simulink model "sf_cdplayer"  (Simulink 7.6)
settings: Solver=FixedStepDiscrete  StartTime=0.0  StopTime=inf  FixedStep=1  RelTol=1e-3
PreLoadFcn:
  | defaultRadioRequestMode = RadioRequestMode.OFF;
  | defaultCdRequestMode = CdRequestMode.EMPTY;
StartFcn:
  | clear sfcdplayerhelper;
  | sfcdplayergui;
StopFcn:
  | delete(sfcdplayergui);
model workspace (MATLAB code in the model file):
  | Ts = 0.01;  % setup system sample rate
settings Model: Creator=The MathWorks Inc.
settings DataIOCC: SaveOutput=off  SaveTime=off
settings OptimizationCC: InlineParams=on  StateBitsets=on  DataBitsets=on  ZeroExternalMemoryAtStartup=off  ZeroInternalMemoryAtStartup=off  InitFltsAndDblsToZero=on  EfficientFloat2IntCast=on  EfficientMapNaN2IntZero=off  OptimizeModelRefInitCode=on  LifeSpan=1
settings DebuggingCC: SolverPrmCheckMsg=none  StrictBusMsg=Warning
settings HardwareCC: ProdIntDivRoundTo=Zero  ProdEndianess=LittleEndian  ProdHWDeviceType=NEC->V850
settings ModelReferenceCC: ModelReferenceNumInstancesAllowed=Single
settings SFSimCC: SimParseCustomCode=off
settings RTWCC: SystemTargetFile=ert.tlc  GenCodeOnly=on  TemplateMakefile=ert_default_tmf  Description=Real-Time Workshop Embedded Coder (no auto configuration)  GenerateReport=on  ProcessScript=ert_make_rtw_hook  IncludeHyperlinkInReport=on  LaunchReport=on  GenerateTraceInfo=on  GenerateTraceReport=on  GenerateTraceReportSl=on  GenerateTraceReportSf=on  GenerateTraceReportEml=on
settings CodeAppCC: IgnoreCustomStorageClasses=off
settings ERTTargetCC: MultiwordLength=2048  GenerateSampleERTMain=on  IncludeMdlTerminateFcn=off  SupportAbsoluteTime=off  SupportNonFinite=off  SupportComplex=off  PurelyIntegerCode=on  ERTCustomFileTemplate=example_file_process.tlc  ConvertIfToSwitch=off  EnableUserReplacementTypes=on
settings ConfigComp: Description=Design Verifier Custom Configuration Component  DVMaxProcessTime=600  DVDisplayUnsatisfiableObjectives=on  DVAutomaticStubbing=off  DVParameters=on  DVModelCoverageObjectives=MCDC  DVMaxTestCaseSteps=500  DVTestSuiteOptimization=CombinedObjectives  DVSaveHarnessModel=on  DVModelReferenceHarness=on  DVSaveReport=on

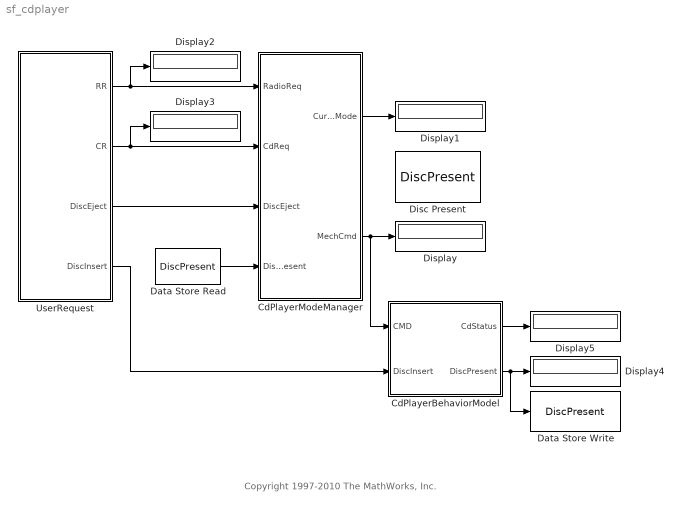
== system sf_cdplayer ==
  note: Copyright 1997-2010 The MathWorks, Inc.
  CdPlayerBehaviorModel : Stateflow chart  TreatAsAtomicUnit=on
  CdPlayerModeManager : Stateflow chart  TreatAsAtomicUnit=on
  Data Store Read : DataStoreRead  DataStoreName=DiscPresent  SampleTime=0
  Data Store Write : DataStoreWrite  DataStoreName=DiscPresent
  Disc Present : DataStoreMemory  DataStoreName=DiscPresent
  Display{,1..5} (6 alike) : Display
  UserRequest : Stateflow chart  TreatAsAtomicUnit=on
  wires:
  UserRequest/2(CR) -> CdPlayerModeManager/2(CdReq), Display3/1
  Data Store Read/1 -> CdPlayerModeManager/4(DiscPresent)
  CdPlayerModeManager/2(MechCmd) -> Display/1, CdPlayerBehaviorModel/1(CMD)
  CdPlayerModeManager/1(CurrentRadioMode) -> Display1/1
  UserRequest/1(RR) -> CdPlayerModeManager/1(RadioReq), Display2/1
  CdPlayerBehaviorModel/1(CdStatus) -> Display5/1
  CdPlayerBehaviorModel/2(DiscPresent) -> Data Store Write/1, Display4/1
  UserRequest/4(DiscInsert) -> CdPlayerBehaviorModel/2(DiscInsert)
  UserRequest/3(DiscEject) -> CdPlayerModeManager/3(DiscEject)

== stateflow chart CdPlayerModeManager ==
  state Eject
    entry:
    MechCmd = EJECT;
  state ModeManager
    (history)
    state ON
      (history)
      state FMMode
        entry:
        CurrentRadioMode = FM;
        MechCmd = STOP;
      state CDMode
        en:
        CurrentRadioMode = CD;
        MechCmd = STOP;
        ex: MechCmd = STOP;
        state Play
          state FastForward
            entry: MechCmd = FF;
          state Rew
            entry: MechCmd = REW;
          state Normal
            entry: MechCmd = PLAY;
          Play -> FastForward [order 1] : [CdReq == FF && !in(FastForward)]
          (default) -> Normal
          Play -> Rew [order 2] : [CdReq == REW && !in(Rew)]
          Play -> Normal [order 3] : [CdReq == PLAY && !in(Normal)]
        state Stop
          entry: MechCmd = STOP;
        (default) -> Stop [order 2]
        (default) -> Play [order 1] : [DiscPresent]
        Play -> Stop [order 1] : [CdReq==STOP]
        Stop -> Play : [DiscPresent && CdReq==PLAY]
      state AMMode
        entry:
        CurrentRadioMode = AM;
        MechCmd = STOP;
      (junction 17) -> AMMode [order 1] : [RadioReq==AM]
      (junction 15) -> FMMode : /*RadioReq==FM*/
      (junction 16) -> CDMode [order 1] : [RadioReq==CD]
      (junction 16) -> (junction 17) [order 2]
      (junction 17) -> (junction 15) [order 2]
      (default) -> (junction 16)
      ON -> (junction 16) [order 1] : [hasChanged(RadioReq)]
    state Standby
      entry: CurrentRadioMode = OFF;
      MechCmd = STOP;
    (default) -> Standby
    Standby -> ON : [RadioReq != OFF]
    ON -> Standby [order 1] : [RadioReq == OFF]
  ModeManager -> Eject : [DiscEject]
  Eject -> ModeManager
  (default) -> ModeManager
  data: RadioReq input Enum: RadioRequestMode =0xFF; CdReq input Enum: CdRequestMode; DiscEject input double; CurrentRadioMode output Enum: RadioRequestMode; DiscPresent input boolean; MechCmd output Enum: CdRequestMode

== stateflow chart UserRequest ==
  (default) -> (junction 49) : {
      | RR = RadioRequestMode(ml.sfcdplayerhelper('get_radio_request'));
      | CR = CdRequestMode(ml.sfcdplayerhelper('get_cd_request'));
      | DiscInsert = ml.sfcdplayerhelper('get_insert_disc');
      | DiscEject = ml.sfcdplayerhelper('get_eject_disc');
      | }
  (junction 49) -> (junction 50)
  data: RR output Enum: RadioRequestMode; CR output Enum: CdRequestMode; DiscEject output boolean; DiscInsert output boolean

== stateflow chart CdPlayerBehaviorModel ==
  state Empty
    CdStatus = EMPTY;
  state Inserting
    CdStatus = DISCINSERT;
  state DiscPresent
    state STOP
      CdStatus = STOP;
    state PLAY
      CdStatus = PLAY;
    state FF
      CdStatus = FF;
    state REW
      CdStatus = REW;
    DiscPresent -> STOP [order 1] : [CMD == STOP]
    DiscPresent -> PLAY [order 2] : [CMD == PLAY]
    (default) -> STOP
    DiscPresent -> FF [order 4] : [CMD == FF]
    DiscPresent -> REW [order 3] : [CMD == REW]
  state Ejecting
    CdStatus = EJECT;
  (default) -> Empty
  Empty -> Inserting : [DiscInsert]
  Inserting -> DiscPresent : [after(1/Ts, tick)]
  DiscPresent -> Ejecting [order 1] : [CMD == EJECT]
  Ejecting -> Empty : [after(1/Ts, tick)]
  data: CMD input double; CdStatus output Enum: CdRequestMode; DiscInsert input boolean; Ts parameter double; DiscPresent output boolean
